simulink model "simulation_regulation"  (Simulink 7.0)
settings: Solver=ode45  StartTime=0.0  StopTime=Temps_Fin  RelTol=1e-3
undefined symbols (not defined in the file or in its folder): bruit_bf, pertu_bf, Rd_tf
libraries: cstblocks x4
settings Model: Creator=adminportog  LastModifiedBy=adminportog

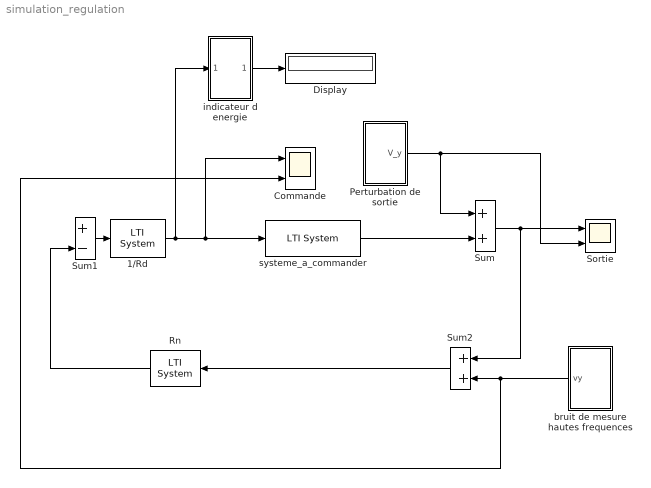
== system simulation_regulation ==
  1/Rd : cstblocks/LTI System  SystemSampleTime=-1  sys=1/Rd_tf  IC=[]
  Commande : Scope  NumInputPorts=2
      settings: TickLabels=on  TimeRange=10  YMin=-2.25~-0.125  YMax=2.5~0.125  MaxDataPoints=50000
  Display : Display
  Perturbation de sortie : Subsystem
  Rn : cstblocks/LTI System  Orientation=left  SystemSampleTime=-1  sys=Rn_tf  IC=[]
  Sortie : Scope  NumInputPorts=2
      settings: TickLabels=on  TimeRange=10  YMin=-5~-5  YMax=5~5  MaxDataPoints=50000
  Sum : Sum  OutDataType=sfix(16)  OutScaling=2^0
  Sum1 : Sum  Inputs=|+-  OutDataType=sfix(16)  OutScaling=2^0
  Sum2 : Sum  Orientation=left  OutDataType=sfix(16)  OutScaling=2^0
  bruit de mesure hautes frequences : Subsystem  Orientation=left
  indicateur d energie : Subsystem
  systeme_a_commander : cstblocks/LTI System  SystemSampleTime=-1  sys=G1  IC=[]
  wires:
  systeme_a_commander/1 -> Sum/2
  Sum/1 -> Sortie/1, Sum2/1
  Sum1/1 -> 1/Rd/1
  1/Rd/1 -> systeme_a_commander/1, Commande/1, indicateur d energie/1(In1)
  Sum2/1 -> Rn/1
  bruit de mesure hautes frequences/1(vy) -> Sum2/2, Commande/2
  Perturbation de sortie/1(V_y) -> Sum/1, Sortie/2
  indicateur d energie/1(Out1) -> Display/1
  Rn/1 -> Sum1/2

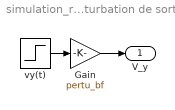
== system simulation_regulation/Perturbation de sortie ==
  Gain : Gain  Gain=pertu_bf  ParameterDataType=sfix(16)  ParameterScaling=2^0  OutDataType=sfix(16)  OutScaling=2^0
  vy(t) : Step  Time=5  SampleTime=0
  V_y : Outport
  wires:
  vy(t)/1 -> Gain/1
  Gain/1 -> V_y/1

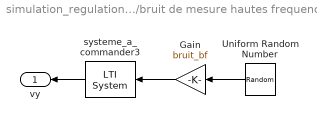
== system simulation_regulation/bruit de mesure hautes frequences ==
  Gain : Gain  Orientation=left  Gain=bruit_bf  ParameterDataType=sfix(16)  ParameterScaling=2^0  OutDataType=sfix(16)  OutScaling=2^0
  Uniform Random Number : UniformRandomNumber  Orientation=left  Minimum=-0.1  Maximum=0.1  SampleTime=0
  systeme_a_commander3 : cstblocks/LTI System  Orientation=left  SystemSampleTime=-1  sys=tf([1 8*1e4],[1 1e5])  IC=[]
  vy : Outport  Orientation=left
  wires:
  Uniform Random Number/1 -> Gain/1
  systeme_a_commander3/1 -> vy/1
  Gain/1 -> systeme_a_commander3/1

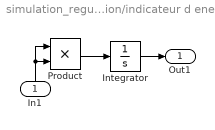
== system simulation_regulation/indicateur d energie ==
  In1 : Inport  Orientation=up
  Integrator : Integrator
  Product : Product  OutDataType=sfix(16)  OutScaling=2^0  RndMeth=Zero
  Out1 : Outport
  wires:
  Product/1 -> Integrator/1
  In1/1 -> Product/2, Product/1
  Integrator/1 -> Out1/1
